simulink model "ex1"  (R2024a)
settings: Solver=FixedStepAuto  StartTime=0.0  StopTime=50  FixedStep=0.001  RelTol=1e-3
values from neighbouring files (symbols this model uses):
  A = [0 1;-5 -1/4]    [ex1_1.m]
  C = [0 1]    [ex1_1.m]
  D = 0    [ex1_1.m]
settings Model: Creator=cosmin  LastModifiedBy=cosmin

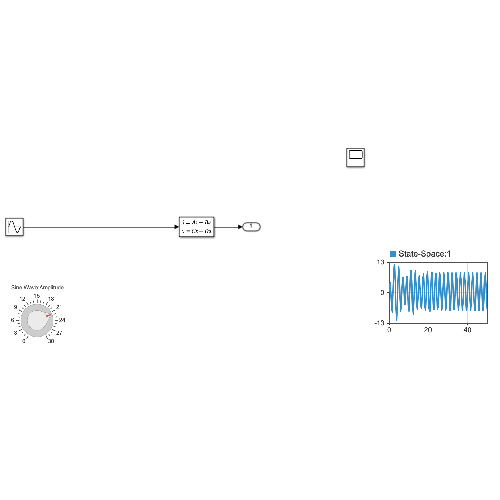
[thumbnail: Simulink's stored preview of the top-level diagram]
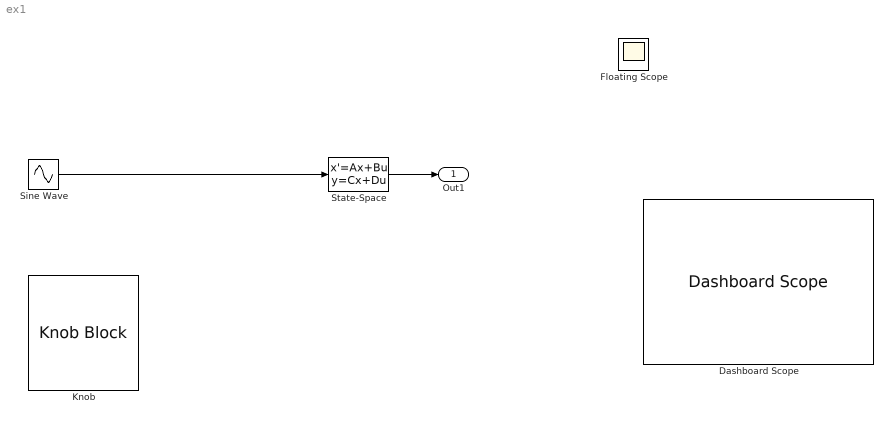
== system ex1 ==
  Dashboard Scope : DashboardScope
  Floating Scope : Scope
      settings: Floating=on
  Knob : KnobBlock  ScaleMax=30
  Sine Wave : Sin  Amplitude=21.60557403564453  Frequency=3  Phase=pi/4  SampleTime=0
  State-Space : StateSpace  A=A  B=B'  C=C  D=D  InitialCondition=0
  Out1 : Outport
  wires:
  Sine Wave/1 -> State-Space/1
  State-Space/1 -> Out1/1
